simulink library "csc_fcv_filter_convergence_lib"  (R2014b)
settings: Solver=ode45  SolverMode=SingleTasking  StartTime=0.0  StopTime=10.0  RelTol=1e-3
undefined symbols (not defined in the file or in its folder): kfl_n_state
libraries: util_info_lib x1, csu_fec_filter_error_check_lib x1
settings Model: Creator=escrane  LastModifiedBy=mstewart

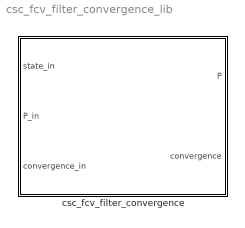
== system csc_fcv_filter_convergence_lib ==
  csc_fcv_filter_convergence : Subsystem

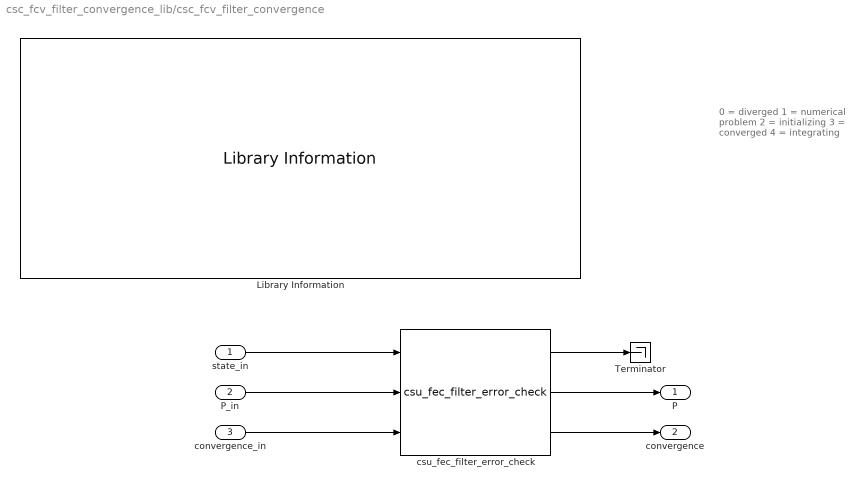
== system csc_fcv_filter_convergence_lib/csc_fcv_filter_convergence ==
  note: 0 = diverged
      | 1 = numerical problem
      | 2 = initializing
      | 3 = converged
      | 4 = integrating
  state_in : Inport
  P_in : Inport  Port=2
  convergence_in : Inport  Port=3
  Library Information : util_info_lib/Library Information  owner='escrane'
  Terminator : Terminator
  csu_fec_filter_error_check : csu_fec_filter_error_check_lib/csu_fec_filter_error_check
  P : Outport  InitialOutput=zeros(kfl_n_state, kfl_n_state)
  convergence : Outport  Port=2  InitialOutput=zeros(kfl_n_state, kfl_n_state)
  wires:
  state_in/1 -> csu_fec_filter_error_check/1
  P_in/1 -> csu_fec_filter_error_check/2
  convergence_in/1 -> csu_fec_filter_error_check/3
  csu_fec_filter_error_check/3 -> convergence/1
  csu_fec_filter_error_check/2 -> P/1
  csu_fec_filter_error_check/1 -> Terminator/1
